simulink model "AsteroidImpact"  (R2023a)
settings: Solver=ode4  StartTime=0.0  StopTime=75  FixedStep=0.1  RelTol=1e-3
settings Model: Creator=KNMALE002  LastModifiedBy=justm
settings SolverCC: AlgebraicLoopSolver=TrustRegion
settings DataIOCC: SaveOutput=off  SignalLogging=off  DSMLogging=off  ReturnWorkspaceOutputs=off  TimeSaveName=simulation_time
settings DebuggingCC: UnconnectedInputMsg=warning  UnconnectedOutputMsg=warning  UnconnectedLineMsg=warning  ArithmeticOperatorsInVariantConditions=warning
settings ModelReferenceCC: EnableRefExpFcnMdlSchedulingChecks=on
settings SFSimCC: CustomCodeUndefinedFunction=UseInterfaceOnly

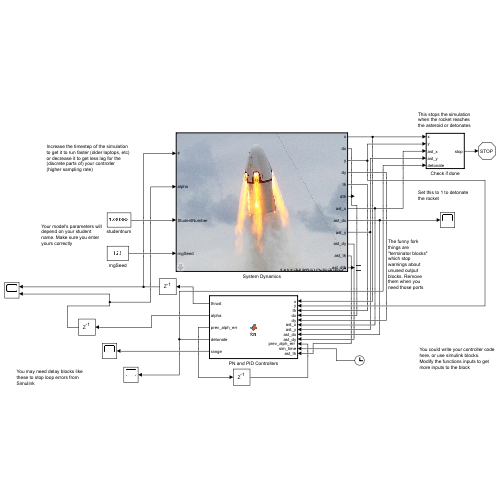
[thumbnail: Simulink's stored preview of the top-level diagram]
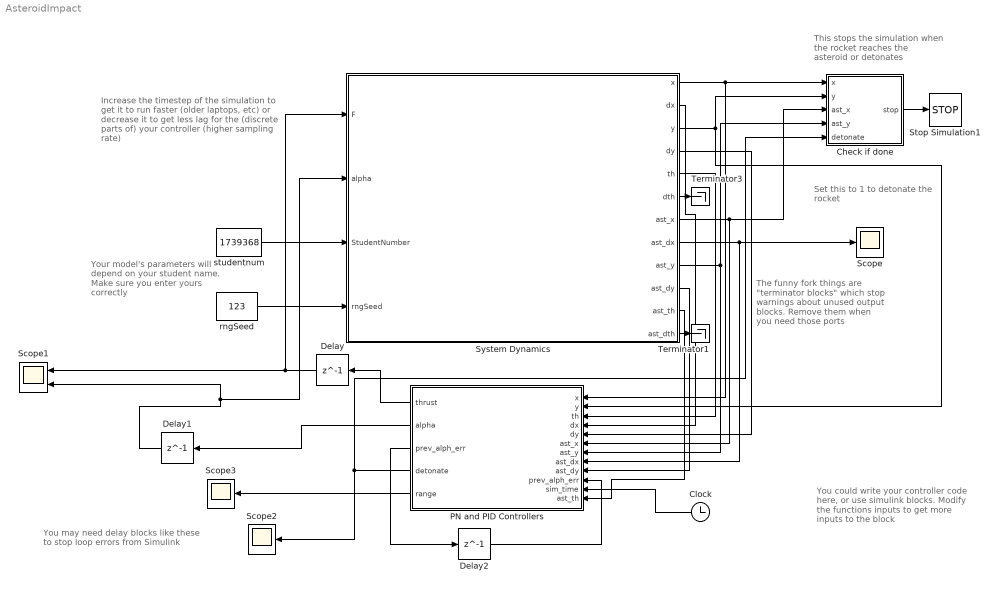
== system AsteroidImpact ==
  note: Increase the timestep of the simulation to get it to run faster (older laptops, etc) or decrease it to get less lag for the (discrete parts of) your controller (higher sampling rate)
  note: You may need delay blocks like these to stop loop errors from Simulink
  note: Your model's parameters will depend on your student name. Make sure you enter yours correctly
  note: You could write your controller code here, or use simulink blocks. Modify the functions inputs to get more inputs to the block
  note: The funny fork things are "terminator blocks" which stop warnings about unused output blocks. Remove them when you need those ports
  note: This stops the simulation when the rocket reaches the asteroid or detonates
  note: Set this to 1 to detonate the rocket
  Check if done : MATLAB Function  TreatAsAtomicUnit=on
  Clock : Clock
  Delay : Delay  DelayLength=1  InitialCondition=10000000000
  Delay1 : Delay  DelayLength=1
  Delay2 : Delay  DelayLength=1  InitialCondition=0
  PN and PID Controllers : MATLAB Function  TreatAsAtomicUnit=on
  Scope : Scope
  Scope1 : Scope  NumInputPorts=2
  Scope2 : Scope
  Scope3 : Scope
  Stop Simulation1 : Stop
  System Dynamics : Subsystem  TreatAsAtomicUnit=on  mask{Value=3}
      mask prompts: Value "Enter mode (1, 2 or 3)"
      mask TypeOptions Value: ScenarioVar/Value
      mask Display: image('lander.jpg');
  Terminator1 : Terminator
  Terminator3 : Terminator
  rngSeed : Constant  Value=123
  studentnum : Constant  Value=1739368
  wires:
  studentnum/1 -> System Dynamics/3(StudentNumber)
  System Dynamics/1(x) -> PN and PID Controllers/1(x), Check if done/1(x)
  rngSeed/1 -> System Dynamics/4(rngSeed)
  System Dynamics/3(y) -> Check if done/2(y), PN and PID Controllers/2(y)
  System Dynamics/7(ast_x) -> Check if done/3(ast_x), PN and PID Controllers/6(ast_x)
  System Dynamics/9(ast_y) -> PN and PID Controllers/7(ast_y), Check if done/4(ast_y)
  System Dynamics/8(ast_dx) -> PN and PID Controllers/8(ast_dx), Scope/1
  System Dynamics/11(ast_th) -> PN and PID Controllers/12(ast_th)
  Check if done/1(stop) -> Stop Simulation1/1
  Delay1/1 -> System Dynamics/2(alpha), Scope1/2
  Delay/1 -> Scope1/1, System Dynamics/1(F)
  PN and PID Controllers/1(thrust) -> Delay/1
  System Dynamics/10(ast_dy) -> PN and PID Controllers/9(ast_dy)
  System Dynamics/5(th) -> PN and PID Controllers/3(th)
  System Dynamics/2(dx) -> PN and PID Controllers/4(dx)
  System Dynamics/4(dy) -> PN and PID Controllers/5(dy)
  PN and PID Controllers/2(alpha) -> Delay1/1
  Delay2/1 -> PN and PID Controllers/10("prev_alph_err ")
  System Dynamics/6(dth) -> Terminator3/1
  Clock/1 -> PN and PID Controllers/11(sim_time)
  PN and PID Controllers/3(prev_alph_err) -> Delay2/1
  PN and PID Controllers/5(range) -> Scope3/1
  PN and PID Controllers/4(detonate) -> Scope2/1, Check if done/5(detonate)
  System Dynamics/12(ast_dth) -> Terminator1/1

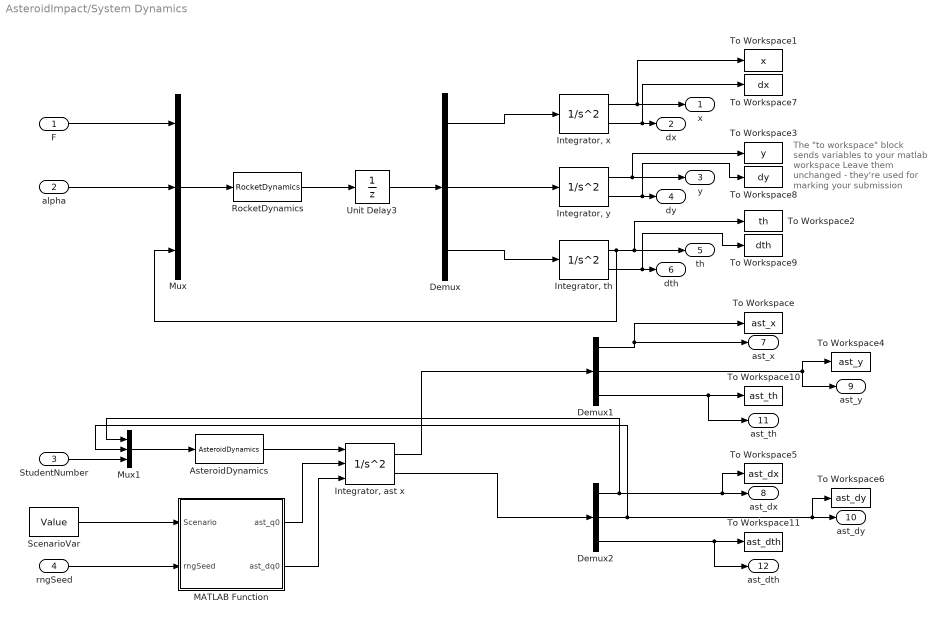
== system AsteroidImpact/System Dynamics ==
  note: The "to workspace" block sends variables to your matlab workspace
      |
      | Leave them unchanged - they're used for marking your submission
  F : Inport
  alpha : Inport  Port=2
  StudentNumber : Inport  Port=3
  rngSeed : Inport  Port=4
  AsteroidDynamics : MATLABFcn  MATLABFcn=AsteroidDynamics  OutputDimensions=3
  Demux : Demux  Outputs=3
  Demux1 : Demux  Outputs=3
  Demux2 : Demux  Outputs=3
  "Integrator, th" : SecondOrderIntegrator  ICX=0  ICDXDT=0
  "Integrator, x" : SecondOrderIntegrator  ICX=0
  "Integrator, y" : SecondOrderIntegrator  ICX=0
  "Integrator, ast x" : SecondOrderIntegrator  ICSourceX=external  ICX=x0  ICSourceDXDT=external
  MATLAB Function : MATLAB Function  TreatAsAtomicUnit=on
  Mux : Mux  Inputs=3
  Mux1 : Mux  Inputs=3
  RocketDynamics : MATLABFcn  MATLABFcn=RocketDynamics  Output1D=off
  ScenarioVar : Constant  Value=Value
  To Workspace : ToWorkspace  VariableName=ast_x  SampleTime=-1
  To Workspace1 : ToWorkspace  VariableName=x  SampleTime=-1
  To Workspace10 : ToWorkspace  VariableName=ast_th  SampleTime=-1
  To Workspace11 : ToWorkspace  VariableName=ast_dth  SampleTime=-1
  To Workspace2 : ToWorkspace  VariableName=th  SampleTime=-1
  To Workspace3 : ToWorkspace  VariableName=y  SampleTime=-1
  To Workspace4 : ToWorkspace  VariableName=ast_y  SampleTime=-1
  To Workspace5 : ToWorkspace  VariableName=ast_dx  SampleTime=-1
  To Workspace6 : ToWorkspace  VariableName=ast_dy  SampleTime=-1
  To Workspace7 : ToWorkspace  VariableName=dx  SampleTime=-1
  To Workspace8 : ToWorkspace  VariableName=dy  SampleTime=-1
  To Workspace9 : ToWorkspace  VariableName=dth  SampleTime=-1
  Unit Delay3 : UnitDelay  SampleTime=-1  HasFrameUpgradeWarning=on
  x : Outport  PortDimensions=1  VectorParamsAs1DForOutWhenUnconnected=off
  dx : Outport  Port=2  PortDimensions=1  VectorParamsAs1DForOutWhenUnconnected=off
  y : Outport  Port=3  PortDimensions=1  VectorParamsAs1DForOutWhenUnconnected=off
  dy : Outport  Port=4  PortDimensions=1  VectorParamsAs1DForOutWhenUnconnected=off
  th : Outport  Port=5  PortDimensions=1  VectorParamsAs1DForOutWhenUnconnected=off
  dth : Outport  Port=6  PortDimensions=1  VectorParamsAs1DForOutWhenUnconnected=off
  ast_x : Outport  Port=7  PortDimensions=1  VectorParamsAs1DForOutWhenUnconnected=off
  ast_dx : Outport  Port=8  PortDimensions=1  VectorParamsAs1DForOutWhenUnconnected=off
  ast_y : Outport  Port=9  PortDimensions=1  VectorParamsAs1DForOutWhenUnconnected=off
  ast_dy : Outport  Port=10  PortDimensions=1  VectorParamsAs1DForOutWhenUnconnected=off
  ast_th : Outport  Port=11  PortDimensions=1  VectorParamsAs1DForOutWhenUnconnected=off
  ast_dth : Outport  Port=12  PortDimensions=1  VectorParamsAs1DForOutWhenUnconnected=off
  wires:
  "Integrator, th"/1 -> th/1, To Workspace2/1, Mux/3
  Demux/1 -> "Integrator, x"/1
  Demux/2 -> "Integrator, y"/1
  Demux/3 -> "Integrator, th"/1
  "Integrator, x"/1 -> x/1, To Workspace1/1
  "Integrator, x"/2 -> To Workspace7/1, dx/1
  "Integrator, y"/2 -> To Workspace8/1, dy/1
  "Integrator, th"/2 -> To Workspace9/1, dth/1
  Mux/1 -> RocketDynamics/1
  RocketDynamics/1 -> Unit Delay3/1
  rngSeed/1 -> MATLAB Function/2(rngSeed)
  ScenarioVar/1 -> MATLAB Function/1(Scenario)
  F/1 -> Mux/1
  alpha/1 -> Mux/2
  Demux1/2 -> To Workspace4/1, ast_y/1
  Demux1/3 -> To Workspace10/1, ast_th/1
  Demux2/3 -> ast_dth/1, To Workspace11/1
  Mux1/1 -> AsteroidDynamics/1
  AsteroidDynamics/1 -> "Integrator, ast x"/1
  "Integrator, ast x"/1 -> Demux1/1
  "Integrator, ast x"/2 -> Demux2/1
  Demux1/1 -> To Workspace/1, ast_x/1
  Demux2/1 -> Mux1/1, To Workspace5/1, ast_dx/1
  Demux2/2 -> Mux1/2, To Workspace6/1, ast_dy/1
  MATLAB Function/1(ast_q0) -> "Integrator, ast x"/2
  MATLAB Function/2(ast_dq0) -> "Integrator, ast x"/3
  StudentNumber/1 -> Mux1/3
  Unit Delay3/1 -> Demux/1
  "Integrator, y"/1 -> y/1, To Workspace3/1

== matlab function AsteroidImpact/System Dynamics/MATLAB Function ==
  data: ast_q0 output; ast_dq0 output; Scenario input; rngSeed input
function [ast_q0, ast_dq0] = fcn(Scenario, rngSeed)
rng(rngSeed);

if (Scenario == 1)
    x0 = -3000;
    y0 =  5000;
    th0 =   0;
    dx0 = 182;
    dy0 = 0;
    dth0 = 0;

elseif (Scenario == 2)
    x0 = -2000 + rand_within_plus_minus(100);
    y0 = 4000 + rand_within_plus_minus(100); 
    th0 = 0;
    dx0 = 170;
    dy0 = 0;
    dth0 = 0.1;

elseif (Scenario == 3)
    x0 = -2500;
    y0 = 3000;
    th0 = 0;
    dx0 = 160;
    dy0 = 100;
    dth0 = deg2rad(rand_within_plus_minus(20)); % rad/sec

else
    error('You entered an invalid mode -- make sure Scenario = 1, 2 or 3')
end

ast_q0  = [ x0;  y0;  th0];
ast_dq0 = [dx0; dy0; dth0];

end

% calling rand_within_plus_minus(100) returns a number between -100 and 100
function n = rand_within_plus_minus(interval)
    n = (rand - 0.5) * 2 * interval;
end

== matlab function AsteroidImpact/PN and PID Controllers ==
  settings: updateMethod=DISCRETE
  data: x input; thrust output; alpha output; y input; th input; dx input; dy input; ast_x input; ast_y input; ast_dx input; ast_dy input; prev_alph_err input; prev_alph_err output; detonate output; range output; sim_time input; ast_th input
function [thrust, alpha, prev_alph_err, detonate, range] = fcn(x, y, th, dx, dy, ast_x, ast_y, ast_dx, ast_dy, prev_alph_err, sim_time, ast_th)

% Constants
mass = 1000; % Mass of the rocket (kg)
gravity = 9.81; % Gravitational acceleration (m/s^2)

% Positions and velocities in inertial frame
rocket_pos = [x; y; 0];    % Rocket's position in 3D
rocket_vel = [dx; dy; 0];  % Rocket's velocity in 3D
asteroid_pos = [ast_x; ast_y; 0];   % Asteroid's position in 3D
asteroid_vel = [ast_dx; ast_dy; 0]; % Asteroid's velocity in 3D

% Persistent variable to lock the chosen arc
persistent chosen_arc
if isempty(chosen_arc)
    chosen_arc = '';
end

% Calculate relative angle of rocket to asteroid
pos_rel = asteroid_pos - rocket_pos;  % Relative position of asteroid w.r.t. rocket
rel_angle = atan2(pos_rel(2), pos_rel(1));  % Angle of rocket relative to asteroid
angle_diff = rel_angle - ast_th;  % Angle relative to asteroid's orientation
angle_diff = mod(angle_diff + pi, 2*pi) - pi;  % Normalize to [-pi, pi]

% Define the center of the front and back arcs
front_arc_center = 0;  % 0 degrees (front face)
back_arc_center = pi;  % 180 degrees (back face)

% Lock the arc when within 1000 meters
range = norm(pos_rel(1:2));  % Range to asteroid center for arc locking
if isempty(chosen_arc) || range > 1000
    front_dist = abs(mod(angle_diff - front_arc_center + pi, 2*pi) - pi);
    back_dist = abs(mod(angle_diff - back_arc_center + pi, 2*pi) - pi);
    if front_dist <= back_dist * 1.3  % Bias toward front arc (1.3x threshold)
        chosen_arc = 'front';
    else
        chosen_arc = 'back';
    end
end

% Set target angle based on locked arc
if strcmp(chosen_arc, 'front')
    target_angle = ast_th + front_arc_center;  % Aim for front arc
else
    target_angle = ast_th + back_arc_center;  % Aim for back arc
end

% Select target impact point within desired arcs
% Base offset distance for impact point
base_offset_distance = 100; % Distance from asteroid center to target point

% Adjust offset distance in terminal phase
if range < 200
    offset_distance = 0; % Aim directly at asteroid surface in terminal phase
else
    offset_distance = base_offset_distance;
end

% Compute target impact point (offset from asteroid center)
target_offset = offset_distance * [cos(target_angle); sin(target_angle); 0];
target_pos = asteroid_pos + target_offset;  % Target point in inertial frame

% Position and velocity of rocket relative to target point
pos_rel = target_pos - rocket_pos;  % Relative position of target w.r.t. rocket
vel_rel = asteroid_vel - rocket_vel;  % Relative velocity (assume asteroid velocity applies to target point)

% Line-of-sight (LOS) calculations:
range = norm(pos_rel(1:2));  % Range to target point in XY-plane
range = max(range, 1); % Prevent division-by-zero in LOS rate
los_rate = (pos_rel(1)*vel_rel(2) - pos_rel(2)*vel_rel(1)) / (range^2);  % Rate of change of LOS angle

% Closing velocity (along LOS direction):
closing_speed = -dot(vel_rel(1:2), pos_rel(1:2)) / range;  % Negative dot product
closing_speed = max(closing_speed, 0.1); % Ensure minimum closing speed for guidance

% Proportional Navigation guidance to intercept the target point
if range < 1500
    nav_gain = 4 + 2 * (1500 - range) / 1350; % Linearly increase from 4 to 6 (1500m to 150m)
    nav_gain = min(max(nav_gain, 4), 6); % Clamp to [4, 6]
else
    nav_gain = 4; % Standard gain for responsiveness
end
normal_accel = nav_gain * closing_speed * los_rate;  % Normal acceleration needed

% Desired acceleration in inertial frame (along the line of sight)
los_dir = pos_rel(1:2) / range;  % Direction vector along the line of sight
perp_dir = [-los_dir(2); los_dir(1)];  % Perpendicular direction vector
desired_accel = normal_accel * perp_dir;  % Desired acceleration in perpendicular direction

% Total acceleration
total_accel = desired_accel + [0; gravity];  % Total acceleration including gravity

% Force in the inertial frame (F = m * a)
force_inertial = mass * [total_accel; 0];  % Force in the inertial frame

% Convert force from inertial frame to body frame
rot_inertial_to_body = transpose(Rotz(th));  % Rotation matrix from world to body frame
force_body = rot_inertial_to_body * force_inertial;  % Force in the rocket's body frame

% Output thrust and angle
% Adjust thrust multiplier based on range to asteroid
if range > 2000
    thrust_multiplier = 1.15; % Higher thrust for initial corrections
elseif range > 1000
    thrust_multiplier = 1.0; % Moderate thrust for mid-range
else
    thrust_multiplier = 0.9; % Lower thrust for terminal phase precision
end
thrust = thrust_multiplier * norm(force_body);  % Thrust magnitude
desired_angle = atan2(force_body(2), force_body(1));  % Desired angle of the thrust vector

% Persistent variable to store the integral term for PID controller
persistent integral_storage
if isempty(integral_storage)
    integral_storage = 0;
end

% PID controller gains
Kp_alph = 0.001;  % Proportional gain
Ki_alph = 0.00001; % Integral gain
Kd_alph = 0.0002;  % Derivative gain

% PID error calculation
alph_err = desired_angle - th;  % The error in the desired thrust angle
integral_storage = integral_storage + alph_err * sim_time;  % Accumulate the integral of the error
alph_int = integral_storage;  % Integral term for the PID controller
alph_deriv = (alph_err - prev_alph_err) / sim_time;  % Derivative term

% PID control equation
control_eq = Kp_alph * alph_err + Ki_alph * alph_int + Kd_alph * alph_deriv;  % Control signal to adjust angle

% Update previous error for the next step
prev_alph_err = alph_err;

% Adjust rocket angle to match selected arc in terminal phase
if sim_time < 6  % Keep vertical launch for the first 6 seconds
    alpha = 0; % Force rocket to fly vertically
elseif range < 1500
    % Blend PID control with arc-aligned angle for smooth transition
    blend_factor = (1500 - range) / 1350; % Linear blend from 0 (1500m) to 1 (150m)
    blend_factor = min(max(blend_factor, 0), 1); % Clamp to [0, 1]
    arc_aligned_angle = target_angle - th; % Angle to align with arc center
    arc_aligned_angle = mod(arc_aligned_angle + pi, 2*pi) - pi; % Normalize to [-pi, pi]
    alpha = (1 - blend_factor) * control_eq + blend_factor * arc_aligned_angle; % Blended angle
    % Add angle error feedback in terminal phase
    if range < 500
        arc_error = mod(angle_diff - front_arc_center + pi, 2*pi) - pi; % For front arc
        if strcmp(chosen_arc, 'back')
            arc_error = mod(angle_diff - back_arc_center + pi, 2*pi) - pi;
        end
        alpha = alpha + 0.05 * arc_error; % Small correction
    end
    alpha = min(max(alpha, -pi/5), pi/5); % Saturate to ±36 degrees
else
    alpha = min(max(control_eq, -pi/6), pi/6);  % PID control with ±30 degrees
end

% Detonation logic
% Check if the rocket is within 150 meters and approaching from valid angles
if range <= 150
    % Compute relative position between rocket and asteroid
    rel_pos = rocket_pos(1:2) - asteroid_pos(1:2);  % Relative position in XY-plane

    % Compute angle of approach (angle from asteroid to rocket)
    approach_angle = atan2(rel_pos(2), rel_pos(1));  % In radians
    approach_angle_deg = rad2deg(approach_angle);    % Convert to degrees

    % Asteroid's orientation angle in degrees
    asteroid_angle_deg = rad2deg(ast_th);

    % Compute angle difference (error in approach angle relative to asteroid's heading)
    angle_error = wrapTo180(approach_angle_deg - asteroid_angle_deg);

    % Detonation conditions:
    % Allow detonation if rocket is within ±30° of asteroid's front (0°)
    % or within ±30° of its back (180°)
    if abs(angle_error) <= 30 || abs(wrapTo180(angle_error - 180)) <= 30
        detonate = 1;  % Valid detonation angle
    else
        detonate = 0;  % Unsafe or ineffective detonation angle
    end
else
    detonate = 0;  % Too far to detonate
end
end

% Function to rotate coordinates around the Z-axis
function A = Rotz(th)
    A = [cos(th)   -sin(th) 0;...  
         sin(th)  cos(th) 0;...
         0        0        1]; 
end

== matlab function AsteroidImpact/Check if done ==
  data: x input; stop output; y input; ast_x input; ast_y input; detonate input
function stop = fcn(x, y, ast_x, ast_y, detonate)
    % given the signal to detonate
    if detonate == 1
        stop = 1;

    % rocket has hit the asteroid
    % adjusted collision distance to increase angle correction time
    elseif norm([x; y] - [ast_x; ast_y]) < 10
        stop = 1;
    
    % rocket has hit the ground OR asteroid is close to they city
    elseif y < 0 || ast_y < 200
        stop = 1;
    
    else
        stop = 0;
    end
end
